simulink model "example"  (R2022b)
settings: Solver=FixedStepAuto  StartTime=0.0  StopTime=inf  FixedStep=0.01  RelTol=1e-3
model workspace (MAT data in the model file):
  vesc_device = internal.Serialport
libraries: instrumentseriallib x3
settings Model: Creator=mkoehler  LastModifiedBy=mkoehler

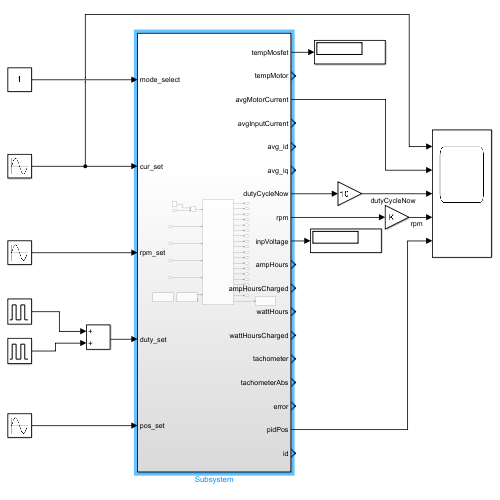
[thumbnail: Simulink's stored preview of the top-level diagram]
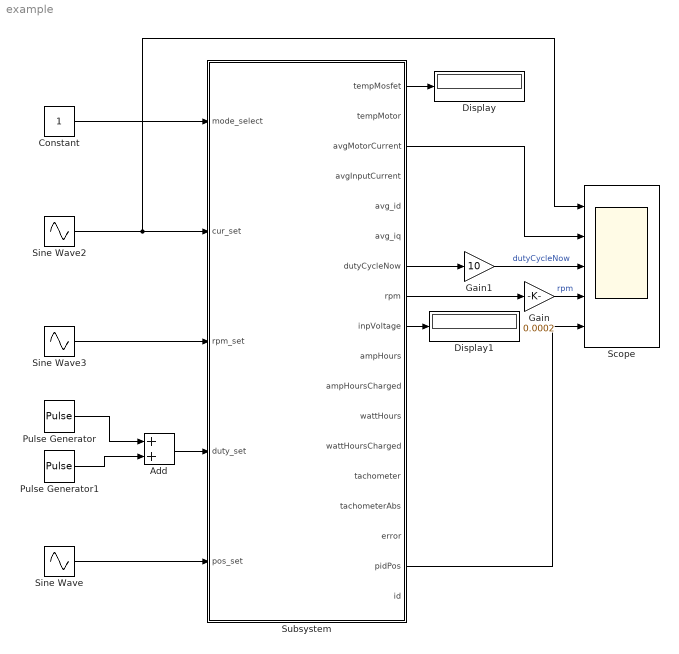
== system example ==
  Add : Sum
  Constant : Constant
  Display : Display
  Display1 : Display
  Gain : Gain  Gain=0.0002
  Gain1 : Gain  Gain=10
  Pulse Generator : DiscretePulseGenerator  PulseType=Time based  Amplitude=-.25  PulseWidth=50  PhaseDelay=1
  Pulse Generator1 : DiscretePulseGenerator  PulseType=Time based  Amplitude=.25  PulseWidth=50
  Scope : Scope  NumInputPorts=5
  Sine Wave : Sin  Amplitude=180  Bias=180  SampleTime=0
  Sine Wave2 : Sin  Amplitude=3  Frequency=8  SampleTime=0
  Sine Wave3 : Sin  Amplitude=2500  Frequency=3  SampleTime=0
  Subsystem : Subsystem
  wires:
  Sine Wave/1 -> Subsystem/5(pos_set)
  Sine Wave3/1 -> Subsystem/3(rpm_set)
  Constant/1 -> Subsystem/1(mode_select)
  Subsystem/1(tempMosfet) -> Display/1
  Pulse Generator1/1 -> Add/2
  Pulse Generator/1 -> Add/1
  Add/1 -> Subsystem/4(duty_set)
  Subsystem/3(avgMotorCurrent) -> Scope/2
  Subsystem/8(rpm) -> Gain/1
  Gain/1 -> Scope/4  "rpm"
  Subsystem/7(dutyCycleNow) -> Gain1/1
  Sine Wave2/1 -> Subsystem/2(cur_set), Scope/1
  Gain1/1 -> Scope/3  "dutyCycleNow"
  Subsystem/17(pidPos) -> Scope/5
  Subsystem/9(inpVoltage) -> Display1/1

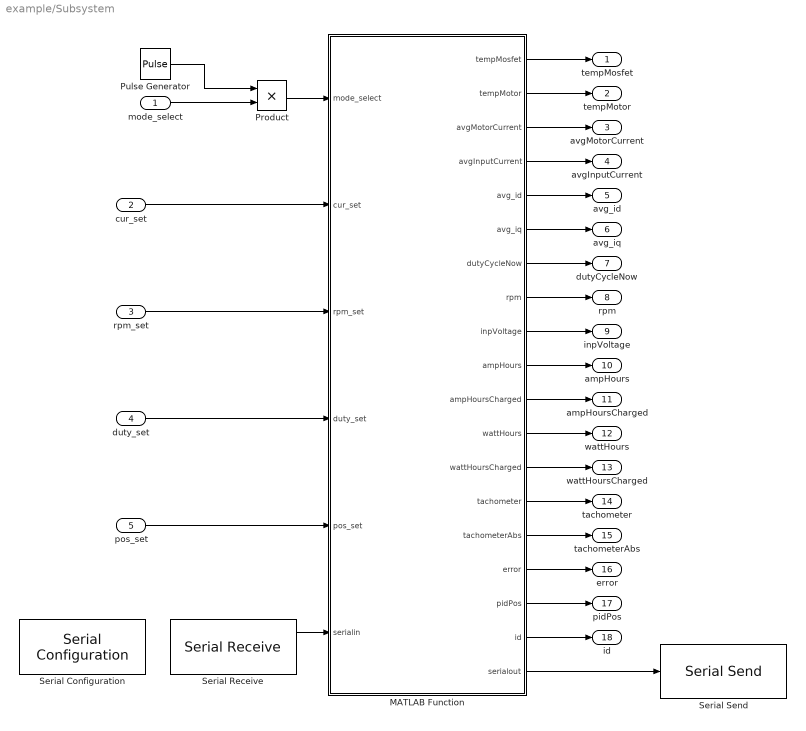
== system example/Subsystem ==
  mode_select : Inport
  cur_set : Inport  Port=2
  rpm_set : Inport  Port=3
  duty_set : Inport  Port=4
  pos_set : Inport  Port=5
  MATLAB Function : MATLAB Function  LoadFcn=|  TreatAsAtomicUnit=on
      | simulink_get_rt_data.m;
      | simulink_req_rt_data.m;
      | simulink_keep_alive.m;
      | simulink_set_current.m;
      | simulink_set_duty.m;
      | simulink_set_pos.m;
      | simulink_set_rpm.m;
  Product : Product
  Pulse Generator : DiscretePulseGenerator  PulseType=Time based  Period=0.02  PulseWidth=50
  Serial Configuration : instrumentseriallib/Serial Configuration  Priority=-200000  PortSel=COM4  Port=COM4  ComPort=COM4  BaudRate=115200  DataBits=8  Parity=none  StopBits=1  ByteOrder=little-endian  FlowControl=none  Timeout=10  SimulateUsing=Interpreted execution  BlockInModel=on  aMode=1
  Serial Receive : instrumentseriallib/Serial Receive  Priority=1  PortSel=COM4  Port=COM4  ComPort=COM4  DataType=uint8  SaveDataType=uint8  ToggleHeader=off  Header=[]  ToggleTerminator=off  Terminator=<none>  CustomTerminator=[]  InputFormat=Column major  ToggleDataSize=on  DataSize=[1 79]  EnableBlockingMode=off  ActionDataUnavailable=Output last received value  ActionWhenDataUnavailable=Output last received value  CustomValue=0  SampleTime=-1  SimulateUsing=Interpreted execution  BlockInModel=on  aMode=1
  Serial Send : instrumentseriallib/Serial Send  Priority=1  PortSel=COM4  Port=COM4  ComPort=COM4  Header=[]  Terminator=<none>  CustomTerminator=[]  EnableBlockingMode=off  SimulateUsing=Interpreted execution  BlockInModel=on  aMode=1
  tempMosfet : Outport
  tempMotor : Outport  Port=2
  avgMotorCurrent : Outport  Port=3
  avgInputCurrent : Outport  Port=4
  avg_id : Outport  Port=5
  avg_iq : Outport  Port=6
  dutyCycleNow : Outport  Port=7
  rpm : Outport  Port=8
  inpVoltage : Outport  Port=9
  ampHours : Outport  Port=10
  ampHoursCharged : Outport  Port=11
  wattHours : Outport  Port=12
  wattHoursCharged : Outport  Port=13
  tachometer : Outport  Port=14
  tachometerAbs : Outport  Port=15
  error : Outport  Port=16
  pidPos : Outport  Port=17
  id : Outport  Port=18
  wires:
  MATLAB Function/2(tempMotor) -> tempMotor/1
  MATLAB Function/4(avgInputCurrent) -> avgInputCurrent/1
  duty_set/1 -> MATLAB Function/4(duty_set)
  MATLAB Function/15(tachometerAbs) -> tachometerAbs/1
  MATLAB Function/6(avg_iq) -> avg_iq/1
  MATLAB Function/5(avg_id) -> avg_id/1
  pos_set/1 -> MATLAB Function/5(pos_set)
  MATLAB Function/13(wattHoursCharged) -> wattHoursCharged/1
  MATLAB Function/8(rpm) -> rpm/1
  MATLAB Function/7(dutyCycleNow) -> dutyCycleNow/1
  Serial Receive/1 -> MATLAB Function/6(serialin)
  MATLAB Function/9(inpVoltage) -> inpVoltage/1
  rpm_set/1 -> MATLAB Function/3(rpm_set)
  MATLAB Function/14(tachometer) -> tachometer/1
  MATLAB Function/12(wattHours) -> wattHours/1
  MATLAB Function/16(error) -> error/1
  MATLAB Function/10(ampHours) -> ampHours/1
  cur_set/1 -> MATLAB Function/2(cur_set)
  MATLAB Function/1(tempMosfet) -> tempMosfet/1
  MATLAB Function/17(pidPos) -> pidPos/1
  MATLAB Function/11(ampHoursCharged) -> ampHoursCharged/1
  MATLAB Function/3(avgMotorCurrent) -> avgMotorCurrent/1
  MATLAB Function/18(id) -> id/1
  MATLAB Function/19(serialout) -> Serial Send/1
  Pulse Generator/1 -> Product/1
  Product/1 -> MATLAB Function/1(mode_select)
  mode_select/1 -> Product/2

== matlab function example/Subsystem/MATLAB Function ==
  data: tempMosfet output; tempMotor output; avgMotorCurrent output; avgInputCurrent output; avg_id output; avg_iq output; dutyCycleNow output; rpm output; inpVoltage output; ampHours output; ampHoursCharged output; wattHours output; wattHoursCharged output; tachometer output; tachometerAbs output; error output; pidPos output; id output; mode_select input; cur_set input; rpm_set input; duty_set input; pos_set input; serialin input; serialout output uint8 size=[1,10]
function [tempMosfet,tempMotor,avgMotorCurrent,avgInputCurrent,avg_id,avg_iq,dutyCycleNow,rpm,inpVoltage,ampHours,ampHoursCharged,wattHours,wattHoursCharged,tachometer,tachometerAbs,error,pidPos,id,serialout] = VESC(mode_select, cur_set, rpm_set, duty_set, pos_set, serialin)

[tempMosfet,tempMotor,avgMotorCurrent,avgInputCurrent,avg_id,avg_iq,dutyCycleNow,rpm,inpVoltage,ampHours,ampHoursCharged,wattHours,wattHoursCharged,tachometer,tachometerAbs,error,pidPos,id] = simulink_get_rt_data(serialin);
pause(0.005)
serialout = uint8(simulink_req_rt_data());


switch mode_select

    case 0
    case 1 % current mode
        serialout = uint8(simulink_set_current(cur_set));
    case 2 % rpm mode
        serialout = uint8(simulink_set_rpm(rpm_set));
    case 3 % duty mode
        serialout = uint8(simulink_set_duty(duty_set));
    case 4 % position mode
        serialout = uint8(simulink_set_pos(pos_set));
end

end
